simulink model "wymiennikdyskretny"  (R2013a)
settings: Solver=ode3  StartTime=0.0  StopTime=2000  FixedStep=0.1  RelTol=1e-3
values from neighbouring files (symbols this model uses):
  c = 1000    [komunikacja.m]
  Cw = 4200    [komunikacja.m]
  Cwym = 2700    [komunikacja.m]
  Fzco = Fzco/3600    [komunikacja.m]
  Fzm = -Fzm    [komunikacja.m]
  Kw = 250000    [komunikacja.m]
  Mm = 3000    [komunikacja.m]
  Tpco = -Tpco    [komunikacja.m]
  Tzm = -Tzm    [komunikacja.m]
undefined symbols (not defined in the file or in its folder): DiscIntNeverNeededParam
settings Model: Creator=asia  LastModifiedBy=asia
settings DataIOCC: FinalStateName=wymiennikdyskretnySimState  SaveFinalState=on  SaveCompleteFinalSimState=on

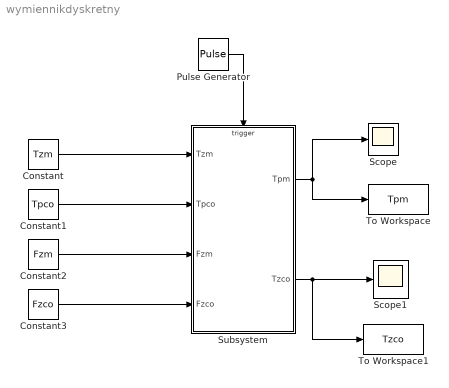
== system wymiennikdyskretny ==
  Constant : Constant  Value=Tzm
  Constant1 : Constant  Value=Tpco
  Constant2 : Constant  Value=Fzm
  Constant3 : Constant  Value=Fzco
  Pulse Generator : DiscretePulseGenerator  PulseType=Time based  PulseWidth=50
  Scope : Scope
  Scope1 : Scope
  Subsystem : Subsystem
  To Workspace : ToWorkspace  VariableName=Tpm  SampleTime=-1
      settings: MaxDataPoints=1
  To Workspace1 : ToWorkspace  VariableName=Tzco  SampleTime=-1
      settings: MaxDataPoints=1
  wires:
  Pulse Generator/1 -> Subsystem/Trigger
  Subsystem/1(Tpm) -> To Workspace/1, Scope/1
  Subsystem/2(Tzco) -> Scope1/1, To Workspace1/1
  Constant/1 -> Subsystem/1(Tzm)
  Constant1/1 -> Subsystem/2(Tpco)
  Constant2/1 -> Subsystem/3(Fzm)
  Constant3/1 -> Subsystem/4(Fzco)

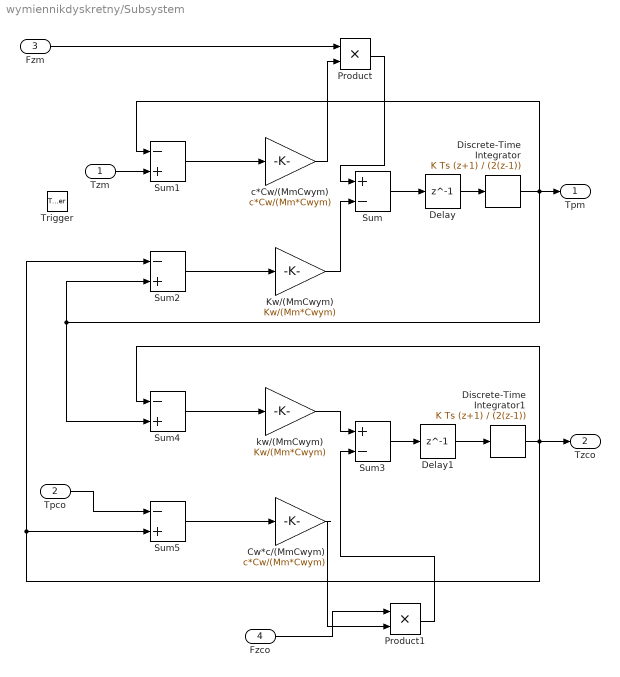
== system wymiennikdyskretny/Subsystem ==
  Tzm : Inport
  Tpco : Inport  Port=2
  Fzm : Inport  Port=3
  Fzco : Inport  Port=4
  Trigger : TriggerPort  PortDimensions=1
  Cw*c/(MmCwym) : Gain  Gain=c*Cw/(Mm*Cwym)
  Delay : Delay  DelayLength=1  InitialCondition=0
  Delay1 : Delay  DelayLength=1  InitialCondition=0
  Discrete-Time Integrator : DiscreteIntegrator  IntegratorMethod=Integration: Trapezoidal  InitialCondition=30  SampleTime=-1  ICPrevOutput=DiscIntNeverNeededParam  ICPrevScaledInput=DiscIntNeverNeededParam
  Discrete-Time Integrator1 : DiscreteIntegrator  IntegratorMethod=Integration: Trapezoidal  InitialCondition=20  SampleTime=-1  ICPrevOutput=DiscIntNeverNeededParam  ICPrevScaledInput=DiscIntNeverNeededParam
  Kw/(MmCwym) : Gain  Gain=Kw/(Mm*Cwym)
  Product : Product
  Product1 : Product
  Sum : Sum  Inputs=+-
  Sum{1..2,4..5} (4 alike) : Sum  Inputs=-+
  Sum3 : Sum  Inputs=+-
  c*Cw/(MmCwym) : Gain  Gain=c*Cw/(Mm*Cwym)
  kw/(MmCwym) : Gain  Gain=Kw/(Mm*Cwym)
  Tpm : Outport  InitialOutput=90
  Tzco : Outport  Port=2  InitialOutput=20
  wires:
  Sum/1 -> Delay/1
  Sum2/1 -> Kw/(MmCwym)/1
  Sum1/1 -> c*Cw/(MmCwym)/1
  c*Cw/(MmCwym)/1 -> Product/2
  Kw/(MmCwym)/1 -> Sum/2
  Tzm/1 -> Sum1/2
  Sum3/1 -> Delay1/1
  Sum5/1 -> Cw*c/(MmCwym)/1
  Sum4/1 -> kw/(MmCwym)/1
  kw/(MmCwym)/1 -> Sum3/1
  Discrete-Time Integrator1/1 -> Tzco/1, Sum2/1, Sum5/2, Sum4/1
  Tpco/1 -> Sum5/1
  Discrete-Time Integrator/1 -> Sum4/2, Sum2/2, Tpm/1, Sum1/1
  Delay/1 -> Discrete-Time Integrator/1
  Delay1/1 -> Discrete-Time Integrator1/1
  Fzm/1 -> Product/1
  Product/1 -> Sum/1
  Fzco/1 -> Product1/1
  Cw*c/(MmCwym)/1 -> Product1/2
  Product1/1 -> Sum3/2
